simulink model "ampel_steuerung_mit_arduirno"  (R2024b)
settings: Solver=FixedStepAuto  StartTime=0.0  StopTime=inf  RelTol=1e-3
libraries: arduinolib x9
settings Model: ExtModeTrigDuration=2  Creator=Steve Kinfack  LastModifiedBy=Steve Kinfack
settings SolverCC: AutoInsertRateTranBlk=on
settings OptimizationCC: EnhancedBackFolding=on  PassReuseOutputArgsAs=Individual arguments  ZeroExternalMemoryAtStartup=off  ZeroInternalMemoryAtStartup=off  MaxStackSize=64  OptimizeBlockOrder=speed  DifferentSizesBufferReuse=on  OptimizationCustomize=off  EfficientTunableParamExpr=on
settings DebuggingCC: ParameterTunabilityLossMsg=error
settings HardwareCC: ProdBitPerInt=16  ProdBitPerPointer=16  ProdBitPerSizeT=16  ProdBitPerPtrDiffT=16  ProdLargestAtomicFloat=None  ProdWordSize=8  ProdHWDeviceType=Atmel->AVR
settings SFSimCC: MATLABDynamicMemAlloc=off
settings RTWCC: Description=Embedded Coder  SystemTargetFile=ert.tlc  HardwareBoard=Arduino Mega 2560  TemplateMakefile=ert_default_tmf  Toolchain=Arduino AVR
settings CodeAppCC: ForceParamTrailComments=on  IgnoreCustomStorageClasses=off  OperatorAnnotations=on  SimulinkDataObjDesc=on  SFDataObjDesc=on  InsertBlockDesc=on
settings ERTTargetCC: SupportContinuousTime=on  SupportVariableSizeSignals=on  ExtModeTransport=3  ExtModeStaticAlloc=on  ExtModeAutomaticAllocSize=off  ExtModeStaticAllocSize=2048  ExtModeMexFile=ext_xcp  ExtModeIntrfLevel=Level2 - Open  InlinedParameterPlacement=Hierarchical

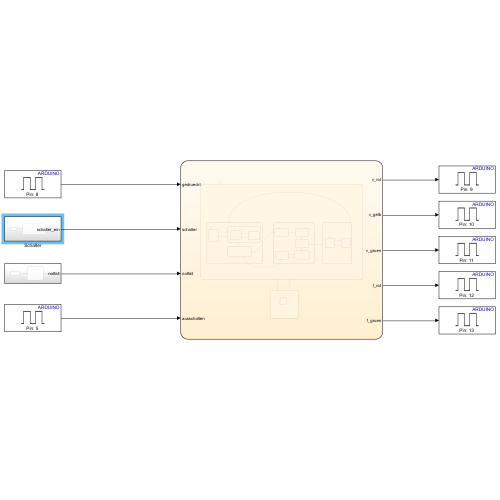
[thumbnail: Simulink's stored preview of the top-level diagram]
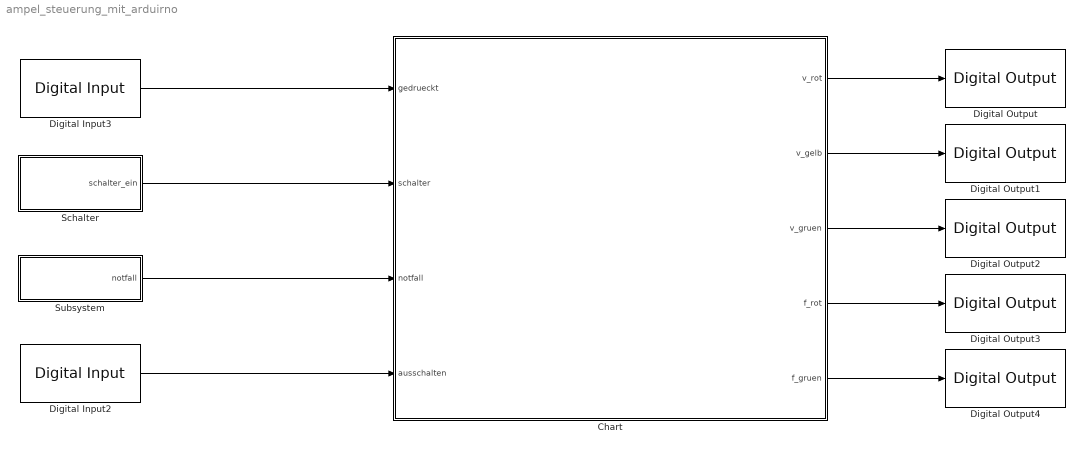
== system ampel_steuerung_mit_arduirno ==
  Chart : Stateflow chart  TreatAsAtomicUnit=on
  Digital Input2 : arduinolib/Digital Input  pinNumber=5  mode=Default  Direction=input  SampleTime=0.1  blockPlatform=arduino
  Digital Input3 : arduinolib/Digital Input  pinNumber=8  mode=Default  Direction=input  SampleTime=0.1  blockPlatform=arduino
  Digital Output : arduinolib/Digital Output  pinNumber=9  Direction=output  blockPlatform=arduino
  Digital Output1 : arduinolib/Digital Output  pinNumber=10  Direction=output  blockPlatform=arduino
  Digital Output2 : arduinolib/Digital Output  pinNumber=11  Direction=output  blockPlatform=arduino
  Digital Output3 : arduinolib/Digital Output  pinNumber=12  Direction=output  blockPlatform=arduino
  Digital Output4 : arduinolib/Digital Output  pinNumber=13  Direction=output  blockPlatform=arduino
  Schalter : Subsystem
  Subsystem : Subsystem
  wires:
  Chart/1(v_rot) -> Digital Output/1
  Chart/2(v_gelb) -> Digital Output1/1
  Chart/3(v_gruen) -> Digital Output2/1
  Chart/4(f_rot) -> Digital Output3/1
  Chart/5(f_gruen) -> Digital Output4/1
  Digital Input2/1 -> Chart/4(ausschalten)
  Digital Input3/1 -> Chart/1(gedrueckt)
  Schalter/1(schalter_ein) -> Chart/2(schalter)
  Subsystem/1(notfall) -> Chart/3(notfall)

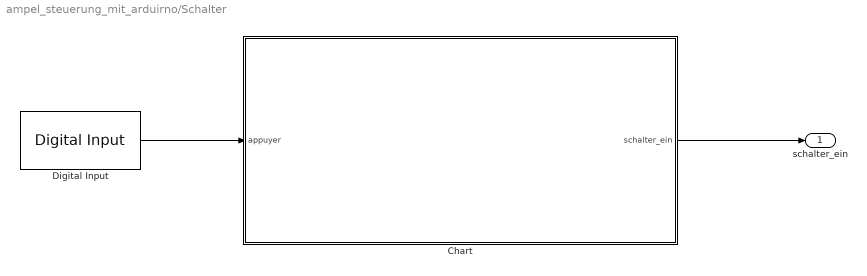
== system ampel_steuerung_mit_arduirno/Schalter ==
  Chart : Stateflow chart  TreatAsAtomicUnit=on
  Digital Input : arduinolib/Digital Input  pinNumber=7  mode=Default  Direction=input  SampleTime=0.1  blockPlatform=arduino
  schalter_ein : Outport
  wires:
  Digital Input/1 -> Chart/1(appuyer)
  Chart/1(schalter_ein) -> schalter_ein/1

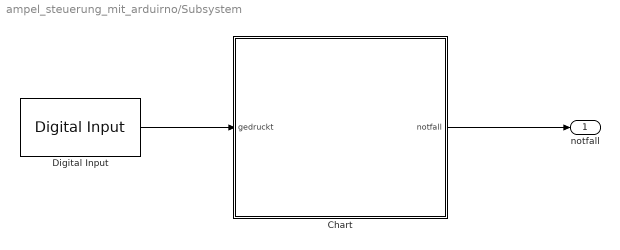
== system ampel_steuerung_mit_arduirno/Subsystem ==
  Chart : Stateflow chart  TreatAsAtomicUnit=on
  Digital Input : arduinolib/Digital Input  pinNumber=6  mode=Default  Direction=input  SampleTime=0.1  blockPlatform=arduino
  notfall : Outport
  wires:
  Digital Input/1 -> Chart/1(gedruckt)
  Chart/1(notfall) -> notfall/1

== stateflow chart ampel_steuerung_mit_arduirno/Schalter/Chart ==
  state schalter_inaktiv
    entry:
    schalter_ein = false;
    exit:
    schalter_ein = true;
  state schalter_aktik
    entry:
    schalter_ein = true;
    exit:
    schalter_ein = false;
  (default) -> schalter_inaktiv
  schalter_inaktiv -> schalter_aktik : [appuyer]
  schalter_aktik -> schalter_inaktiv : [appuyer]
  data: appuyer input; schalter_ein output boolean =false

== stateflow chart ampel_steuerung_mit_arduirno/Subsystem/Chart ==
  state notfall_aus
    entry:
    notfall = false;
    exit:
    notfall = true;
  state notfall_ein
    entry:
    notfall = true;
    exit:
    notfall = false
  (default) -> notfall_aus
  notfall_aus -> notfall_ein : [gedruckt]
  notfall_ein -> notfall_aus : [gedruckt]
  data: gedruckt input; notfall output boolean

== stateflow chart ampel_steuerung_mit_arduirno/Chart ==
  settings: updateMethod=CONTINUOUS
  state Normaler_betrieb
    state Startvorgang
      state A
        state Gelb_blink_und_f_rot
          entry:
          v_gelb = true;
          f_rot = true;
          exit:
          v_gelb = false;
        state Gelb_blink_und_f_rot1
          entry:
          v_gelb = false;
          f_rot = true;
          exit:
          v_gelb = true;
        (default) -> Gelb_blink_und_f_rot
        Gelb_blink_und_f_rot -> Gelb_blink_und_f_rot1 : after(1, sec)
        Gelb_blink_und_f_rot1 -> Gelb_blink_und_f_rot : after(1, sec)
      state Ampel_Aus
        entry:
        v_rot = false;
        v_gelb = false;
        v_gruen = false;
        f_rot = false;
        f_gruen = false;
      state Verkehr_wechsel_von_gelb_auf_rot
        entry:
        v_gelb = false;
        v_rot = true;
      (default) -> Ampel_Aus
      Ampel_Aus -> A : [schalter == 1]
      A -> Ampel_Aus [order 1] : [schalter == 0]
      A -> Verkehr_wechsel_von_gelb_auf_rot [order 2] : after(10, sec)
    state Betrieb
      state F_wechselt_von_gruen_auf_rot
        entry:
        f_gruen = false;
        f_rot = true;
      state F_wechselt_von_rot_auf_gruen
        entry:
        f_rot = false;
        f_gruen = true;
        exit:
        f_gruen = false;
      state V_schaltet_von_rot_auf_rot_gelb
        entry:
        v_rot = true;
        v_gelb = true;
        exit:
        v_rot = false;
        v_gelb = false;
      state V_schaltet_von_rot_gelb_auf_gruen
        entry:
        v_rot = false;
        v_gelb = false;
        v_gruen = true;
        exit:
        v_gruen = false;
      state V_schaltet_von_gruen_auf_gelb
        entry:
        v_gruen = false;
        v_gelb = true;
        exit:
        v_gelb = false;
      (default) -> F_wechselt_von_rot_auf_gruen
      F_wechselt_von_rot_auf_gruen -> F_wechselt_von_gruen_auf_rot : after(15, sec)
      F_wechselt_von_gruen_auf_rot -> V_schaltet_von_rot_auf_rot_gelb : after(2, sec)
      V_schaltet_von_rot_auf_rot_gelb -> V_schaltet_von_rot_gelb_auf_gruen [order 1] : after(2, sec)
      V_schaltet_von_rot_gelb_auf_gruen -> V_schaltet_von_gruen_auf_gelb [order 1] : after(40, sec)
      V_schaltet_von_rot_gelb_auf_gruen -> V_schaltet_von_gruen_auf_gelb [order 2] : after(15, sec)[gedrueckt]
    state Ausschalt_vorgang
      state V_blink_gelb
        entry:
        v_gelb = true;
        exit:
        v_gelb = false;
      state V_blink_gelb1
        entry:
        v_gelb = false;
        exit:
        v_gelb = true;
      (default) -> V_blink_gelb
      V_blink_gelb -> V_blink_gelb1 : after(1, sec)
      V_blink_gelb1 -> V_blink_gelb : after(1, sec)
    Ausschalt_vorgang -> Startvorgang : after(10, sec)
    (default) -> Startvorgang
    Verkehr_wechsel_von_gelb_auf_rot -> F_wechselt_von_rot_auf_gruen : after(5, sec)
    V_schaltet_von_rot_auf_rot_gelb -> Ausschalt_vorgang [order 2] : [ausschalten]
    V_schaltet_von_gruen_auf_gelb -> Verkehr_wechsel_von_gelb_auf_rot : after(2, sec)
  state Notfall
    state emergency
      entry:
      v_rot = true;
      v_gelb = false;
      v_gruen = false;
      f_rot = true;
      f_gruen = false;
  (default) -> Normaler_betrieb
  Normaler_betrieb -> Notfall : [notfall == 1]
  Notfall -> Normaler_betrieb : [notfall == 0]
  data: v_rot output boolean =false; v_gelb output boolean =false; v_gruen output boolean =false; f_rot output boolean =false; f_gruen output boolean =false; gedrueckt input; schalter input; notfall input; ausschalten input
